simulink library "Lib_CanCommunication"  (R2019b)
settings: Solver=VariableStepAuto  StartTime=0.0  StopTime=10.0  RelTol=1e-3
PostLoadFcn:
  | , if any(exist('dsrtsu_mdlpostloadfcn', 'file') == [2, 3, 6]), try dsrtsu_mdlpostloadfcn('Execute', bdroot); catch fprintf('Error in PostLoadFcn (dsrtsu_mdlpostloadfcn) for model "%s":\n %s\n', bdroot, lasterr); end, end,
undefined symbols (not defined in the file): Counter, CRC, default_customer_can_bus, default_vehicle_state_bus, LateralAcceleration, LongitudinalAcceleration, Motion, Powertrain_1, Steering, steering_angle_range_rad_to_steering_wheel_angle_range_deg_gain, SteeringWheelAngle, SteeringWheelAngleSign, SteeringWheelSpeed, SteeringWheelSpeedSign, SteeringWheelTorque, SteeringWheelTorqueSign, VehicleVelocity, YawRate, YawRateSign
libraries: rtican x8, simulink x6
(part 1 of 3)
settings Model: DSRTSU_INTERNAL_RTI_VER=550  DSRTSU_INTERNAL_RTI_TYPE=rti1401  RTICANMMDATA=struct('GeneralSetupData',struct('modelroot','C:\fav\stack\src\autobox\Simulink\Models','generalsettings',struct('filesettings',struct('destfolder',struct('Name','RTICANMM_FILES','Check',1),'buildfolder',struct('Name','.','Check',1),'AbsDestfolder',struct('Name','C:\fav\stack\src\autobox\Simulink\Models\RTICANMM_FILES'),'AbsBuildfolder',struct('Name','C:\fav\stack\src\autobox\Simulink\Models'))),'options',struct('addpaths',1,'rmpaths',1,'addtrcexclusion',logical(1),'cannavigator',struct('checkmonitoring',0),'show_usrtrc',0,'use_usrtrc',0),'advanced',struct('options',[1 1 1 1 1 1 1 1 1 1 1 1 1 1 1 1 1 1 1 1 1 1 1 1 1 1 1 1 1 1 1 1 1 1 1 1 1 1 1 1 1 1 1 1 1 1 1 1 1 1 1 1 1 1 1 1 1 1 1 1 1 1 1 1 1 1 1 1 1 1 1 1 1 1 1 1 1 1 1 1 1 1 1 1 1 1 1 1 1 1 1 1 1 1 1 1 1 1 1 1]),'MPSetup',{{}},'modelname','Lib_CanCommunication','block','Lib_CanCommunication'))  DSRTSU_INTERNAL_RTIFPGA=150  Creator=bernhard  LastModifiedBy=kessler
settings DataIOCC: ReturnWorkspaceOutputs=off
settings DebuggingCC: ArithmeticOperatorsInVariantConditions=warning
settings SFSimCC: SimUseLocalCustomCode=off  CustomCodeUndefinedFunction=UseInterfaceOnly
settings RTWCC: RTWUseLocalCustomCode=off

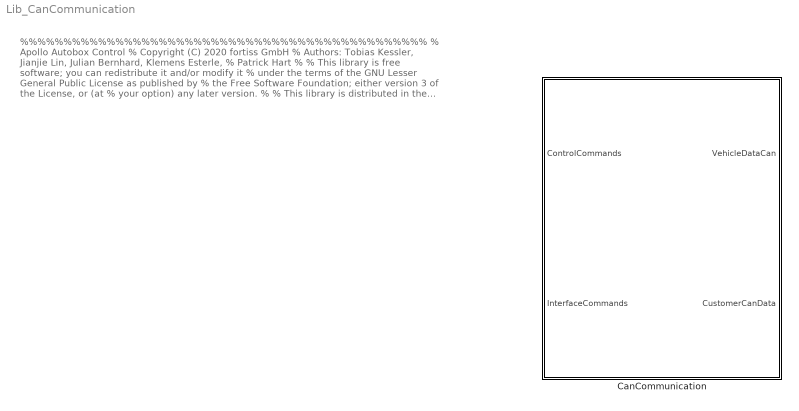
== system Lib_CanCommunication ==
  note: %%%%%%%%%%%%%%%%%%%%%%%%%%%%%%%%%%%%%%%%%%%%%%%
      | % Apollo Autobox Control
      | % Copyright (C) 2020 fortiss GmbH
      | % Authors: Tobias Kessler, Jianjie Lin, Julian Bernhard, Klemens Esterle,
      | % Patrick Hart
      | %
      | % This library is free software; you can redistribute it and/or modify it
      | % under the terms of the GNU Lesser General Public License as published by
      | % the Free Software Foundation; either version 3 of the License, or (at
      | % your option) any later version.
      | %
      | % This library is distributed in the hope that it will be useful, but
      | % WITHOUT ANY WARRANTY; without even the implied warranty of
      | % MERCHANTABILITY or FITNESS FOR A PARTICULAR PURPOSE. See the GNU Lesser
      | % General Public License for more details.
      | %
      | % You should have received a copy of the GNU Lesser General Public License
      | % along with this library; if not, write to the Free Software Foundation,
      | % Inc., 51 Franklin Street, Fifth Floor, Boston, MA 02110-1301, USA.
      | %%%%%%%%%%%%%%%%%%%%%%%%%%%%%%%%%%%%%%%%%%%%%%%
  CanCommunication : Subsystem

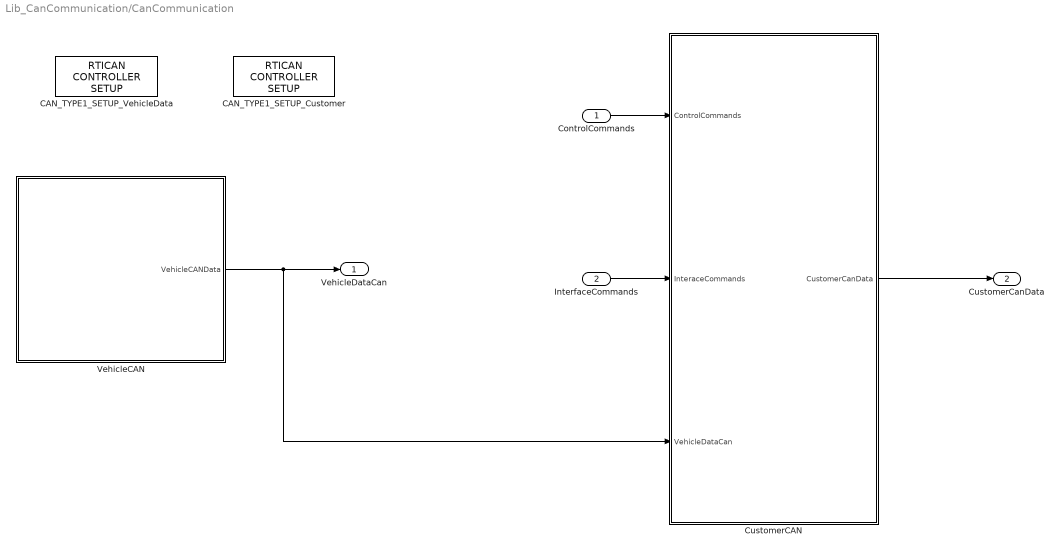
== system Lib_CanCommunication/CanCommunication ==
  ControlCommands : Inport  OutDataTypeStr=Bus: ControlCommands
  InterfaceCommands : Inport  Port=2  OutDataTypeStr=Bus: InterfaceCommands
  CAN_TYPE1_SETUP_Customer : rtican/RTICAN CONTROLLER SETUP   Reserved1=[]  Reserved2=[]  Reserved3=[]  Reserved4=[]  AcceptanceMask=[]  ArbitrationField=[]  Parameters=[]  SFcnRTICANSettings=[]  MS_Struct=[]  BoardTypeNo=[]  BoardNo=[]  ChannelNo=[]  DialogFcn=[]  UnitName=[]  Revision=[]  UnitValues=[]  DSProperties=struct('RTI',struct('Version',uint32(12),'BlockType',struct('isSLSource',uint8(0),'isSLSink',uint8(0),'isHWSource',uint8(0),'isHWSink',uint8(0),'isSetup',uint8(1),'isInline',uint8(1),'isNonInline',uint8(0),'isInterrupt',uint8(0),'isChannelwise',uint8(0)),'IOBoardType','RTICAN','UnitType','NON_MESSAGE','Identifier','MASTER','DialogType','ML','BlockSet','RTICAN','SlaveProcessor','CAN'))  RTIBlockInterface=struct('InputPortsWidth',int32(0),'InputPortsActive',0,'OutputPortsWidth',int32(0),'OutputPortsActive',0,'DialogFcn','rtican_master_setup_gui','BlockDisplay',{{['CAN CONTROLLER\n SETUP'],'center'}},'IconTransparency','on','InitLevel',3,'IWork',{{{'',uint32(2)}}},'BlockName',struct('Token',{{'CAN_TYPE','_SETUP_M','_C'}},'BlockParam',{{'BoardTypeNo','BoardNo','ChannelNo'}}),'ParameterTunableNames',{{}})  RTIBlockParameters="struct('BoardTypeNo',{{1,'OFF',[]}},'BoardNo',{{1,'ON',[1 16]}},'ChannelNo',{{1,'ON',[1 2]}},'AcceptanceMask',{{0,'OFF',[]}},'ArbitrationField',{{0,'OFF',[]}},'Parameters',{{struct('Config',struct('Baudrate',500,'SampleMode',1,'UsedParamSet',1,'validSettings',1,'isBTRvalues',0,'Advanced',struct('Baudrate',{500,500,500},'Frequency',{24000000,36000000,64000000},'Settings',{struct('SMPL',0,'BRP',0,'NBT',24,'TSEG1',15,'TSEG2',6,'SJW',3,'SP',70),struct('SMPL',0,'BRP',1,'NBT',18,'TSEG1',14,'TSEG2',1,'SJW',1,'SP',88),struct('SMPL',0,'BRP',3,'NBT',16,'TSEG1',12,'TSEG2',1,'SJW',1,'SP',87)},'BTR0',{192,65,67},'BTR1',{111,30,28})),'configType',1,'Options',struct('DataFileSelected',1,'DataFileName',{{'..\\dbc\\customer_can_tfd7-17008-03_fortiss_gte.dbc'}},'DataFileDate',{{['02-Aug-2018 13:38:32']}},'InterfaceFcn','rtican_dbc_file_parser','InterfaceFcnFileName','','LabelConfigType','volatile','AcceptanceMaskSelected',0,'MsgDataType','SgnSpecification','NumType','hex','MaskType','STD','AcceptanceMask',0,'ArbitrationField',0,'UseMultipleMessageAccess',1),'RxReceiveStdOptions',struct('RxServiceStdEnabled',0,'RxServiceStdMsgIdent',1000,'RxServiceStdIdentNumType',1,'RxServiceStdIdentMask',0,'RxServiceStdMaskNumType',1,'RxServiceStdQueueSize',64),'RxReceiveXtdOptions',struct('RxServiceXtdEnabled',0,'RxServiceXtdMsgIdent',1001,'RxServiceXtdIdentNumType',1,'RxServiceXtdIdentMask',0,'RxServiceXtdMaskNumType',1,'RxServiceXtdQueueSize',64),'PartialNetworkingOptions',struct('switchedon',0,'format',1,'idmask',['    XXXXX XXXXXXXX XXXXXXXX XXXXXXXX'],'idcode','0','idfilter','0','datamaskused',0,'datalength',1,'datamask','0x0000000000000000','partialnetworkenable',0),'general',struct('Termination_common',2,'Termination_C252',1,'BusConfigurationRegister',0,'Transceiver','ISO11898','isFromLib',0)),'OFF',[]}},'CCPParameters',{{struct('CRO',struct('Format','STD','NumFormat','hex','Id',1639),'DTO',struct('Format','STD','NumFormat','hex','Id',2017),'StationAdr',struct('NumFormat','hex','Value',57),'StationId',struct('Value',['dSPACE CCP Service']),'Enabled',0),'OFF',[]}},'XCPParameters',{{struct('MASTER',struct('Format','STD','NumFormat','hex','Id',256),'SLAVE',struct('Format','STD','NumFormat','hex','Id',510),'Enabled',0,'PIDTransmissionEnabled',0),'OFF',[]}},'GroupId',{{struct('Group',{{'RTICAN'}},'No',2,'Behavior',{{'EVER'}},'BlockType',{{'SOURCE'}},'NameChangeFlag',1),'OFF',[]}},'SFcnRTICANSettings',{{struct('Baudrate',500,'configType',1,'AdvancedConfig',struct('Frequency',{},'BTR0',{},'BTR1',{}),'UsedParamSet',1,'STDMaskSelected','no','XTDMaskSelected','no','BoardType','DS1','BoardNo',1,'ControllerNo',1,'Transceiver','ISO11898','BusConfigRegister',0,'TerminationRes',-1,'UseMultipleMessageAccess','yes','STDRXSrvcUsed','no','STDRXSrvcMsgId',1000,'STDRXSrvcMsgMask',0,'STDRXSrvcQueueSize',64,'XTDRXSrvcUsed','no','XTDRXSrvcMsgId',1001,'XTDRXSrvcQueueSize',64,'XTDRXSrvcMsgMask',0,'PN_IsPNTransciever',0,'PN_IsPNEnabled',0,'PN_MsgFormat',1,'PN_idcode',0,'PN_idmask',2047,'PN_datamaskused',0,'PN_datalength',0,'PN_datamask',['0xFF, 0xFF, 0xFF, 0xFF, 0xFF, 0xFF, 0xFF, 0xFF']),'OFF',[]}},'SFcnRTICCPSettings',{{struct('CRO',struct('Format','STD','NumFormat','hex','Id',1639),'DTO',struct('Format','STD','NumFormat','hex','Id',2017),'StationAdr',struct('NumFormat','hex','Value',57),'StationId',struct('Value',['dSPACE CCP Service']),'Enabled',0),'OFF',[]}},'SFcnRTIXCPSettings',{{struct('MASTER',struct('Format','STD','NumFormat','hex','Id',256),'SLAVE',struct('Format','STD','NumFormat','hex','Id',510),'Enabled',0,'PIDTransmissionEnabled',0),'OFF',[]}},'TLCFileName',{{'rtican_master_setup','OFF',[]}})"  RTISFcnParameters=struct('SFcnRTICANSettings','struct','SFcnRTICCPSettings','struct','SFcnRTIXCPSettings','struct','AcceptanceMask','int32','ArbitrationField','int32','TLCFileName','char')  RTIBlockParaDefault="struct('BoardTypeNo',4302,'BoardNo',1,'ChannelNo',1,'AcceptanceMask',0,'ArbitrationField',0,'Parameters',struct('Config',struct('Baudrate',500,'SampleMode',1,'UsedParamSet',1,'validSettings',1,'isBTRvalues',0,'Advanced',struct('Frequency',16000000,'BTR0',64,'BTR1',28,'Settings',struct('SMPL',0,'BRP',0,'NBT',16,'TSEG1',12,'TSEG2',1,'SJW',1,'SP',87))),'configType',1,'Options',struct('DataFileSelected',0,'DataFileName',{{['<no datafile support>']}},'DataFileDate',{{''}},'InterfaceFcn','rtican_dbc_file_parser','InterfaceFcnFileName','','LabelConfigType','volatile','AcceptanceMaskSelected',0,'MsgDataType','AllwaysDouble','NumType','hex','MaskType','STD','AcceptanceMask',0,'ArbitrationField',0,'UseMultipleMessageAccess',0),'RxReceiveStdOptions',struct('RxServiceStdEnabled',0,'RxServiceStdMsgIdent',1000,'RxServiceStdIdentNumType',1,'RxServiceStdIdentMask',0,'RxServiceStdMaskNumType',1,'RxServiceStdQueueSize',64),'RxReceiveXtdOptions',struct('RxServiceXtdEnabled',0,'RxServiceXtdMsgIdent',1001,'RxServiceXtdIdentNumType',1,'RxServiceXtdIdentMask',0,'RxServiceXtdMaskNumType',1,'RxServiceXtdQueueSize',64),'PartialNetworkingOptions',struct('switchedon',0,'format',1,'idmask',['    XXXXX XXXXXXXX XXXXXXXX XXXXXXXX'],'idcode','0','idfilter','0','datamaskused',0,'datalength',1,'datamask','0x0000000000000000','partialnetworkenable',0),'general',struct('Termination_common',1,'Termination_C252',1,'BusConfigurationRegister',0,'Transceiver','ISO11898','isFromLib',1)),'CCPParameters',struct('CRO',struct('Format','STD','NumFormat','hex','Id',1639),'DTO',struct('Format','STD','NumFormat','hex','Id',2017),'StationAdr',struct('NumFormat','hex','Value',57),'StationId',struct('Value',['dSPACE CCP Service']),'Enabled',0),'XCPParameters',struct('MASTER',struct('Format','STD','NumFormat','hex','Id',256),'SLAVE',struct('Format','STD','NumFormat','hex','Id',510),'Enabled',0,'PIDTransmissionEnabled',0),'GroupId',struct('Group',{{'RTICAN'}},'No',1,'Behavior',{{'EVER'}},'BlockType',{{'SOURCE'}},'NameChangeFlag',1),'SFcnRTICANSettings',struct('Baudrate',500,'configType',1,'AdvandedConfig',struct('Frequency',16000000,'BTR0','0x40','BTR1','0x1C'),'UsedParamSet',1,'STDMaskSelected','no','XTDMaskSelected','no','BoardType','DS4302','BoardNo',1,'ControllerNo',1,'Transceiver','ISO11898','BusConfigRegister',0,'TerminationRes',120,'UseMultipleMessageAccess','no','STDRXSrvcUsed','no','STDRXSrvcMsgId',1000,'STDRXSrvcMsgMask',0,'STDRXSrvcQueueSize',64,'XTDRXSrvcUsed','no','XTDRXSrvcMsgId',1001,'XTDRXSrvcQueueSize',64,'XTDRXSrvcMsgMask',0),'SFcnRTICCPSettings',struct('CRO',struct('Format','STD','NumFormat','hex','Id',1639),'DTO',struct('Format','STD','NumFormat','hex','Id',2017),'StationAdr',struct('NumFormat','hex','Value',57),'StationId',struct('Value',['dSPACE CCP Service']),'Enabled',0),'SFcnRTIXCPSettings',struct('MASTER',struct('Format','STD','NumFormat','hex','Id',256),'SLAVE',struct('Format','STD','NumFormat','hex','Id',510),'Enabled',0,'PIDTransmissionEnabled',0),'TLCFileName','rtican_master_setup')"
      settings: AttributesFormatString=Group Id: RTICAN2\n  SourceProductName=dSPACE RTI CAN Blockset
  CAN_TYPE1_SETUP_VehicleData : rtican/RTICAN CONTROLLER SETUP   Reserved1=[]  Reserved2=[]  Reserved3=[]  Reserved4=[]  AcceptanceMask=[]  ArbitrationField=[]  Parameters=[]  SFcnRTICANSettings=[]  MS_Struct=[]  BoardTypeNo=[]  BoardNo=[]  ChannelNo=[]  DialogFcn=[]  UnitName=[]  Revision=[]  UnitValues=[]  DSProperties=struct('RTI',struct('Version',uint32(12),'BlockType',struct('isSLSource',uint8(0),'isSLSink',uint8(0),'isHWSource',uint8(0),'isHWSink',uint8(0),'isSetup',uint8(1),'isInline',uint8(1),'isNonInline',uint8(0),'isInterrupt',uint8(0),'isChannelwise',uint8(0)),'IOBoardType','RTICAN','UnitType','NON_MESSAGE','Identifier','MASTER','DialogType','ML','BlockSet','RTICAN','SlaveProcessor','CAN'))  RTIBlockInterface=struct('InputPortsWidth',int32(0),'InputPortsActive',0,'OutputPortsWidth',int32(0),'OutputPortsActive',0,'DialogFcn','rtican_master_setup_gui','BlockDisplay',{{['CAN CONTROLLER\n SETUP'],'center'}},'IconTransparency','on','InitLevel',3,'IWork',{{{'',uint32(2)}}},'BlockName',struct('Token',{{'CAN_TYPE','_SETUP_M','_C'}},'BlockParam',{{'BoardTypeNo','BoardNo','ChannelNo'}}),'ParameterTunableNames',{{}})  RTIBlockParameters="struct('BoardTypeNo',{{1,'OFF',[]}},'BoardNo',{{1,'ON',[1 16]}},'ChannelNo',{{2,'ON',[1 2]}},'AcceptanceMask',{{0,'OFF',[]}},'ArbitrationField',{{0,'OFF',[]}},'Parameters',{{struct('Config',struct('Baudrate',500,'SampleMode',1,'UsedParamSet',1,'validSettings',1,'isBTRvalues',0,'Advanced',struct('Baudrate',{500,500,500},'Frequency',{24000000,36000000,64000000},'Settings',{struct('SMPL',0,'BRP',0,'NBT',24,'TSEG1',15,'TSEG2',6,'SJW',3,'SP',70),struct('SMPL',0,'BRP',1,'NBT',18,'TSEG1',14,'TSEG2',1,'SJW',1,'SP',88),struct('SMPL',0,'BRP',3,'NBT',16,'TSEG1',12,'TSEG2',1,'SJW',1,'SP',87)},'BTR0',{192,65,67},'BTR1',{111,30,28})),'configType',1,'Options',struct('DataFileSelected',1,'DataFileName',{{'..\\dbc\\vehicledata_can_tfd7-17008-03_fortiss_gte.dbc'}},'DataFileDate',{{['02-Aug-2018 13:38:32']}},'InterfaceFcn','rtican_dbc_file_parser','InterfaceFcnFileName','','LabelConfigType','volatile','AcceptanceMaskSelected',0,'MsgDataType','SgnSpecification','NumType','hex','MaskType','STD','AcceptanceMask',0,'ArbitrationField',0,'UseMultipleMessageAccess',1),'RxReceiveStdOptions',struct('RxServiceStdEnabled',0,'RxServiceStdMsgIdent',1000,'RxServiceStdIdentNumType',1,'RxServiceStdIdentMask',0,'RxServiceStdMaskNumType',1,'RxServiceStdQueueSize',64),'RxReceiveXtdOptions',struct('RxServiceXtdEnabled',0,'RxServiceXtdMsgIdent',1001,'RxServiceXtdIdentNumType',1,'RxServiceXtdIdentMask',0,'RxServiceXtdMaskNumType',1,'RxServiceXtdQueueSize',64),'PartialNetworkingOptions',struct('switchedon',0,'format',1,'idmask',['    XXXXX XXXXXXXX XXXXXXXX XXXXXXXX'],'idcode','0','idfilter','0','datamaskused',0,'datalength',1,'datamask','0x0000000000000000','partialnetworkenable',0),'general',struct('Termination_common',2,'Termination_C252',1,'BusConfigurationRegister',0,'Transceiver','ISO11898','isFromLib',0)),'OFF',[]}},'CCPParameters',{{struct('CRO',struct('Format','STD','NumFormat','hex','Id',1639),'DTO',struct('Format','STD','NumFormat','hex','Id',2017),'StationAdr',struct('NumFormat','hex','Value',57),'StationId',struct('Value',['dSPACE CCP Service']),'Enabled',0),'OFF',[]}},'XCPParameters',{{struct('MASTER',struct('Format','STD','NumFormat','hex','Id',256),'SLAVE',struct('Format','STD','NumFormat','hex','Id',510),'Enabled',0,'PIDTransmissionEnabled',0),'OFF',[]}},'GroupId',{{struct('Group',{{'RTICAN'}},'No',1,'Behavior',{{'EVER'}},'BlockType',{{'SOURCE'}},'NameChangeFlag',1),'OFF',[]}},'SFcnRTICANSettings',{{struct('Baudrate',500,'configType',1,'AdvancedConfig',struct('Frequency',{},'BTR0',{},'BTR1',{}),'UsedParamSet',1,'STDMaskSelected','no','XTDMaskSelected','no','BoardType','DS1','BoardNo',1,'ControllerNo',2,'Transceiver','ISO11898','BusConfigRegister',0,'TerminationRes',-1,'UseMultipleMessageAccess','yes','STDRXSrvcUsed','no','STDRXSrvcMsgId',1000,'STDRXSrvcMsgMask',0,'STDRXSrvcQueueSize',64,'XTDRXSrvcUsed','no','XTDRXSrvcMsgId',1001,'XTDRXSrvcQueueSize',64,'XTDRXSrvcMsgMask',0,'PN_IsPNTransciever',0,'PN_IsPNEnabled',0,'PN_MsgFormat',1,'PN_idcode',0,'PN_idmask',2047,'PN_datamaskused',0,'PN_datalength',0,'PN_datamask',['0xFF, 0xFF, 0xFF, 0xFF, 0xFF, 0xFF, 0xFF, 0xFF']),'OFF',[]}},'SFcnRTICCPSettings',{{struct('CRO',struct('Format','STD','NumFormat','hex','Id',1639),'DTO',struct('Format','STD','NumFormat','hex','Id',2017),'StationAdr',struct('NumFormat','hex','Value',57),'StationId',struct('Value',['dSPACE CCP Service']),'Enabled',0),'OFF',[]}},'SFcnRTIXCPSettings',{{struct('MASTER',struct('Format','STD','NumFormat','hex','Id',256),'SLAVE',struct('Format','STD','NumFormat','hex','Id',510),'Enabled',0,'PIDTransmissionEnabled',0),'OFF',[]}},'TLCFileName',{{'rtican_master_setup','OFF',[]}})"  RTISFcnParameters=struct('SFcnRTICANSettings','struct','SFcnRTICCPSettings','struct','SFcnRTIXCPSettings','struct','AcceptanceMask','int32','ArbitrationField','int32','TLCFileName','char')  RTIBlockParaDefault="struct('BoardTypeNo',4302,'BoardNo',1,'ChannelNo',1,'AcceptanceMask',0,'ArbitrationField',0,'Parameters',struct('Config',struct('Baudrate',500,'SampleMode',1,'UsedParamSet',1,'validSettings',1,'isBTRvalues',0,'Advanced',struct('Frequency',16000000,'BTR0',64,'BTR1',28,'Settings',struct('SMPL',0,'BRP',0,'NBT',16,'TSEG1',12,'TSEG2',1,'SJW',1,'SP',87))),'configType',1,'Options',struct('DataFileSelected',0,'DataFileName',{{['<no datafile support>']}},'DataFileDate',{{''}},'InterfaceFcn','rtican_dbc_file_parser','InterfaceFcnFileName','','LabelConfigType','volatile','AcceptanceMaskSelected',0,'MsgDataType','AllwaysDouble','NumType','hex','MaskType','STD','AcceptanceMask',0,'ArbitrationField',0,'UseMultipleMessageAccess',0),'RxReceiveStdOptions',struct('RxServiceStdEnabled',0,'RxServiceStdMsgIdent',1000,'RxServiceStdIdentNumType',1,'RxServiceStdIdentMask',0,'RxServiceStdMaskNumType',1,'RxServiceStdQueueSize',64),'RxReceiveXtdOptions',struct('RxServiceXtdEnabled',0,'RxServiceXtdMsgIdent',1001,'RxServiceXtdIdentNumType',1,'RxServiceXtdIdentMask',0,'RxServiceXtdMaskNumType',1,'RxServiceXtdQueueSize',64),'PartialNetworkingOptions',struct('switchedon',0,'format',1,'idmask',['    XXXXX XXXXXXXX XXXXXXXX XXXXXXXX'],'idcode','0','idfilter','0','datamaskused',0,'datalength',1,'datamask','0x0000000000000000','partialnetworkenable',0),'general',struct('Termination_common',1,'Termination_C252',1,'BusConfigurationRegister',0,'Transceiver','ISO11898','isFromLib',1)),'CCPParameters',struct('CRO',struct('Format','STD','NumFormat','hex','Id',1639),'DTO',struct('Format','STD','NumFormat','hex','Id',2017),'StationAdr',struct('NumFormat','hex','Value',57),'StationId',struct('Value',['dSPACE CCP Service']),'Enabled',0),'XCPParameters',struct('MASTER',struct('Format','STD','NumFormat','hex','Id',256),'SLAVE',struct('Format','STD','NumFormat','hex','Id',510),'Enabled',0,'PIDTransmissionEnabled',0),'GroupId',struct('Group',{{'RTICAN'}},'No',1,'Behavior',{{'EVER'}},'BlockType',{{'SOURCE'}},'NameChangeFlag',1),'SFcnRTICANSettings',struct('Baudrate',500,'configType',1,'AdvandedConfig',struct('Frequency',16000000,'BTR0','0x40','BTR1','0x1C'),'UsedParamSet',1,'STDMaskSelected','no','XTDMaskSelected','no','BoardType','DS4302','BoardNo',1,'ControllerNo',1,'Transceiver','ISO11898','BusConfigRegister',0,'TerminationRes',120,'UseMultipleMessageAccess','no','STDRXSrvcUsed','no','STDRXSrvcMsgId',1000,'STDRXSrvcMsgMask',0,'STDRXSrvcQueueSize',64,'XTDRXSrvcUsed','no','XTDRXSrvcMsgId',1001,'XTDRXSrvcQueueSize',64,'XTDRXSrvcMsgMask',0),'SFcnRTICCPSettings',struct('CRO',struct('Format','STD','NumFormat','hex','Id',1639),'DTO',struct('Format','STD','NumFormat','hex','Id',2017),'StationAdr',struct('NumFormat','hex','Value',57),'StationId',struct('Value',['dSPACE CCP Service']),'Enabled',0),'SFcnRTIXCPSettings',struct('MASTER',struct('Format','STD','NumFormat','hex','Id',256),'SLAVE',struct('Format','STD','NumFormat','hex','Id',510),'Enabled',0,'PIDTransmissionEnabled',0),'TLCFileName','rtican_master_setup')"
      settings: AttributesFormatString=Group Id: RTICAN1\n  SourceProductName=dSPACE RTI CAN Blockset
  CustomerCAN : Subsystem
  VehicleCAN : Subsystem
  VehicleDataCan : Outport  OutDataTypeStr=Bus: vehicle_data_can_bus  VectorParamsAs1DForOutWhenUnconnected=off
  CustomerCanData : Outport  Port=2  OutDataTypeStr=Bus: customer_can_bus  VectorParamsAs1DForOutWhenUnconnected=off
  wires:
  VehicleCAN/1(VehicleCANData) -> VehicleDataCan/1, CustomerCAN/3(VehicleDataCan)
  CustomerCAN/1(CustomerCanData) -> CustomerCanData/1
  ControlCommands/1 -> CustomerCAN/1(ControlCommands)
  InterfaceCommands/1 -> CustomerCAN/2(InteraceCommands)

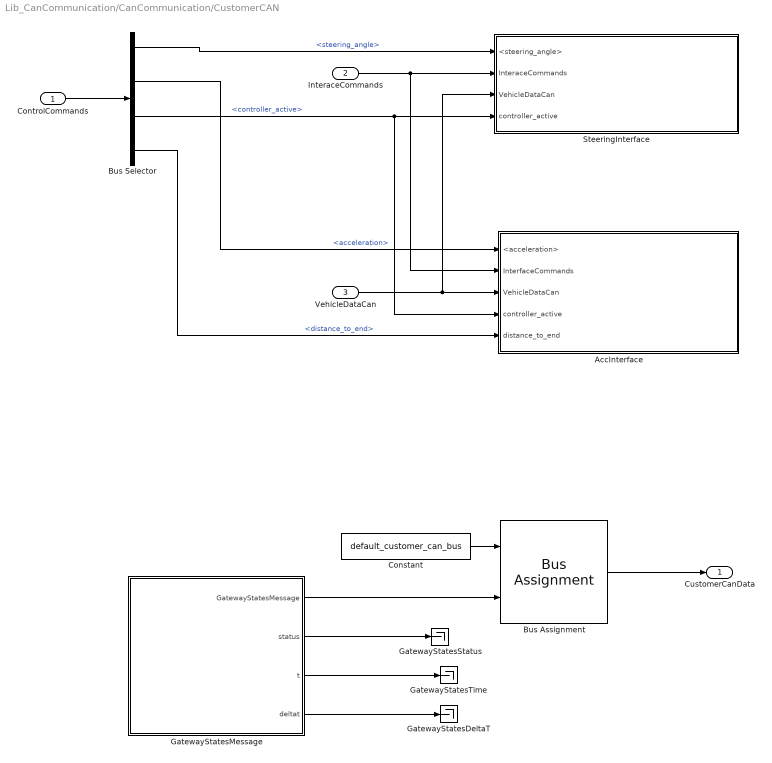
== system Lib_CanCommunication/CanCommunication/CustomerCAN ==
  ControlCommands : Inport  OutDataTypeStr=Bus: ControlCommands
  InteraceCommands : Inport  Port=2  OutDataTypeStr=Bus: InterfaceCommands
  VehicleDataCan : Inport  Port=3
  AccInterface : Subsystem
  Bus Assignment : BusAssignment  AssignedSignals=Gateway_States
  Bus Selector : BusSelector  OutputSignals=steering_angle,acceleration,controller_active,distance_to_end
  Constant : Constant  Value=default_customer_can_bus  OutDataTypeStr=Bus: customer_can_bus
  GatewayStatesDeltaT : Terminator
  GatewayStatesMessage : Subsystem
  GatewayStatesStatus : Terminator
  GatewayStatesTime : Terminator
  SteeringInterface : Subsystem
  CustomerCanData : Outport  VectorParamsAs1DForOutWhenUnconnected=off
  wires:
  Bus Selector/4 -> AccInterface/5(distance_to_end)  "<distance_to_end>"
  Bus Selector/1 -> SteeringInterface/1(<steering_angle>)  "<steering_angle>"
  Bus Selector/2 -> AccInterface/1(<acceleration>)  "<acceleration>"
  Bus Selector/3 -> SteeringInterface/4(controller_active), AccInterface/4(controller_active)  "<controller_active>"
  VehicleDataCan/1 -> AccInterface/3(VehicleDataCan), SteeringInterface/3(VehicleDataCan)
  Constant/1 -> Bus Assignment/1
  Bus Assignment/1 -> CustomerCanData/1
  ControlCommands/1 -> Bus Selector/1
  InteraceCommands/1 -> SteeringInterface/2(InteraceCommands), AccInterface/2(InterfaceCommands)
  GatewayStatesMessage/2(status) -> GatewayStatesStatus/1
  GatewayStatesMessage/3(t) -> GatewayStatesTime/1
  GatewayStatesMessage/4(deltat) -> GatewayStatesDeltaT/1
  GatewayStatesMessage/1(GatewayStatesMessage) -> Bus Assignment/2

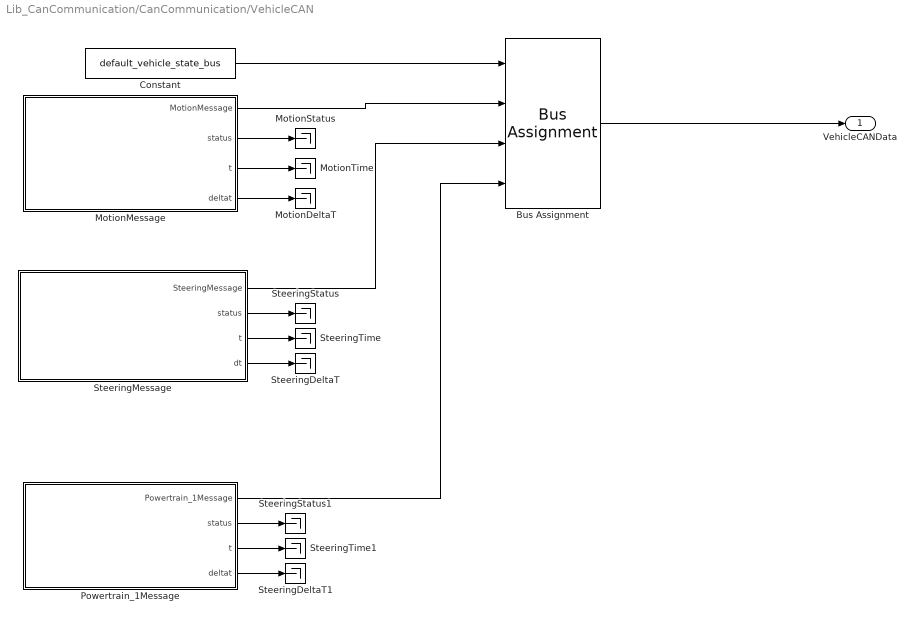
== system Lib_CanCommunication/CanCommunication/VehicleCAN ==
  Bus Assignment : BusAssignment  AssignedSignals=Motion,Steering,Powertrain_1
  Constant : Constant  Value=default_vehicle_state_bus  OutDataTypeStr=Bus: vehicle_data_can_bus
  MotionDeltaT : Terminator
  MotionMessage : Subsystem
  MotionStatus : Terminator
  MotionTime : Terminator
  Powertrain_1Message : Subsystem
  SteeringDeltaT : Terminator
  SteeringDeltaT1 : Terminator
  SteeringMessage : Subsystem
  SteeringStatus : Terminator
  SteeringStatus1 : Terminator
  SteeringTime : Terminator
  SteeringTime1 : Terminator
  VehicleCANData : Outport  VectorParamsAs1DForOutWhenUnconnected=off
  wires:
  Powertrain_1Message/1(Powertrain_1Message) -> Bus Assignment/4
  Powertrain_1Message/4(deltat) -> SteeringDeltaT1/1
  Powertrain_1Message/2(status) -> SteeringStatus1/1
  Powertrain_1Message/3(t) -> SteeringTime1/1
  SteeringMessage/3(t) -> SteeringTime/1
  MotionMessage/2(status) -> MotionStatus/1
  MotionMessage/4(deltat) -> MotionDeltaT/1
  SteeringMessage/2(status) -> SteeringStatus/1
  SteeringMessage/4(dt) -> SteeringDeltaT/1
  MotionMessage/3(t) -> MotionTime/1
  Bus Assignment/1 -> VehicleCANData/1
  MotionMessage/1(MotionMessage) -> Bus Assignment/2
  Constant/1 -> Bus Assignment/1
  SteeringMessage/1(SteeringMessage) -> Bus Assignment/3

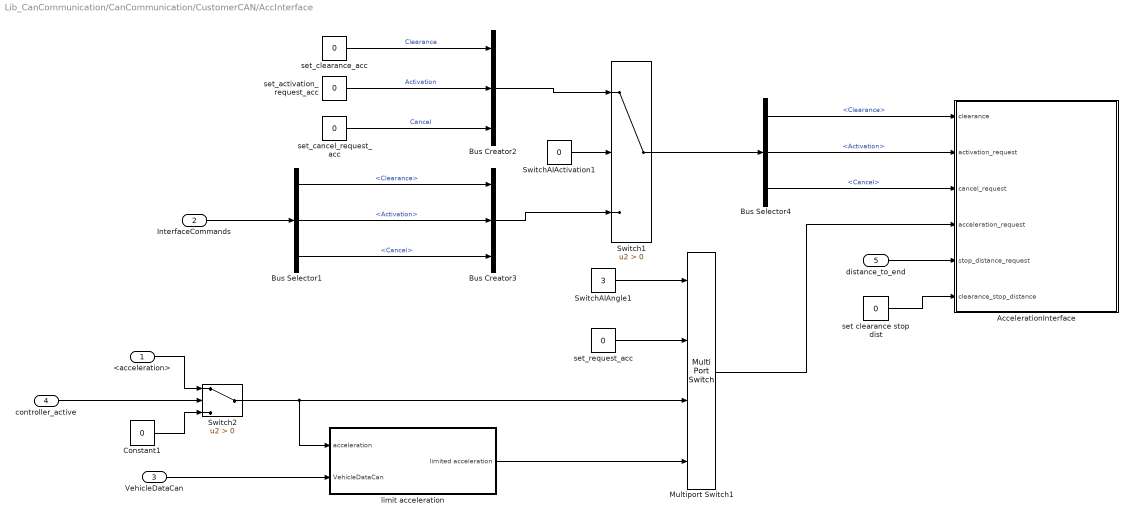
== system Lib_CanCommunication/CanCommunication/CustomerCAN/AccInterface ==
  <acceleration> : Inport
  InterfaceCommands : Inport  Port=2
  VehicleDataCan : Inport  Port=3
  controller_active : Inport  Port=4
  distance_to_end : Inport  Port=5
  AccelerationInterface : Subsystem
  Bus Creator2 : BusCreator  Inputs=3
  Bus Creator3 : BusCreator  Inputs=3
  Bus Selector1 : BusSelector  OutputSignals=AccelerationInterfaceCommands.Clearance,AccelerationInterfaceCommands.Activation,AccelerationInterfaceCommands.Cancel
  Bus Selector4 : BusSelector  OutputSignals=Clearance,Activation,Cancel
  Constant1 : Constant  Value=0
  Multiport Switch1 : MultiPortSwitch
  Switch1 : Switch  Criteria=u2 > Threshold
  Switch2 : Switch  Criteria=u2 > Threshold
  SwitchAIActivation1 : Constant  Value=0
  SwitchAIAngle1 : Constant  Value=3
  limit acceleration : Subsystem
  set clearance stop dist : Constant  Value=0  OutDataTypeStr=boolean
  set_activation_request_acc : Constant  Value=0  OutDataTypeStr=boolean
  set_cancel_request_acc : Constant  Value=0  OutDataTypeStr=boolean
  set_clearance_acc : Constant  Value=0  OutDataTypeStr=boolean
  set_request_acc : Constant  Value=0
  wires:
  set clearance stop dist/1 -> AccelerationInterface/6(clearance_stop_distance)
  distance_to_end/1 -> AccelerationInterface/5(stop_distance_request)
  controller_active/1 -> Switch2/2
  <acceleration>/1 -> Switch2/1
  Constant1/1 -> Switch2/3
  set_request_acc/1 -> Multiport Switch1/2
  Bus Selector1/2 -> Bus Creator3/2  "<Activation>"
  Bus Creator3/1 -> Switch1/3
  set_clearance_acc/1 -> Bus Creator2/1  "Clearance"
  Bus Selector4/3 -> AccelerationInterface/3(cancel_request)  "<Cancel>"
  Bus Selector1/1 -> Bus Creator3/1  "<Clearance>"
  Bus Selector4/1 -> AccelerationInterface/1(clearance)  "<Clearance>"
  Multiport Switch1/1 -> AccelerationInterface/4(acceleration_request)
  SwitchAIActivation1/1 -> Switch1/2
  set_activation_request_acc/1 -> Bus Creator2/2  "Activation"
  Bus Creator2/1 -> Switch1/1
  Bus Selector4/2 -> AccelerationInterface/2(activation_request)  "<Activation>"
  Switch1/1 -> Bus Selector4/1
  Bus Selector1/3 -> Bus Creator3/3  "<Cancel>"
  set_cancel_request_acc/1 -> Bus Creator2/3  "Cancel"
  SwitchAIAngle1/1 -> Multiport Switch1/1
  limit acceleration/1(limited acceleration) -> Multiport Switch1/4
  InterfaceCommands/1 -> Bus Selector1/1
  VehicleDataCan/1 -> limit acceleration/2(VehicleDataCan)
  Switch2/1 -> limit acceleration/1(acceleration), Multiport Switch1/3

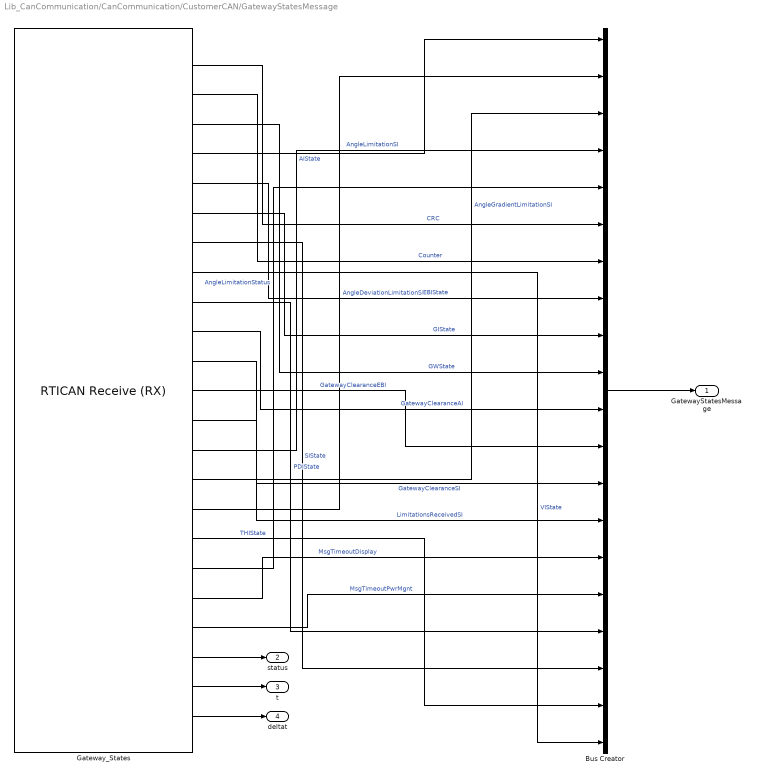
== system Lib_CanCommunication/CanCommunication/CustomerCAN/GatewayStatesMessage ==
  Bus Creator : BusCreator  Inputs=20  OutDataTypeStr=Bus: Gateway_States  NonVirtualBus=on
  Gateway_States : rtican/RTICAN Receive (RX)   Reserved1=[]  Reserved2=[]  Reserved3=[]  Reserved4=[]  SfcnMessage=[]  Msg_Struct=[]  BoardTypeNo=[]  BoardNo=[]  ChannelNo=[]  Parameters=[]  DialogFcn=[]  UnitName=[]  Revision=[]  UnitValues=[]  DSProperties=struct('RTI',struct('Version',uint32(5),'BlockType',struct('isSLSource',uint8(1),'isSLSink',uint8(1),'isHWSource',uint8(0),'isHWSink',uint8(0),'isSetup',uint8(0),'isInline',uint8(1),'isNonInline',uint8(0),'isInterrupt',uint8(0),'isChannelwise',uint8(0)),'IOBoardType','RTICAN','UnitType','MESSAGE','Identifier','RX','DialogType','MSVC','BlockSet','RTICAN','SlaveProcessor','CAN'))  RTIBlockInterface=struct('OutputPortsWidth',int32([1 1 1 1 1 1 1 1 1 1 1 1 1 1 1 1 1 1 1 1 1 1 1]),'OutputPortsActive',ones(1,23),'OutputPortsName',{{'CRC','Counter','GWState','AIState','EBIState','GIState','SIState','VIState','PDIState','GatewayClearanceAI','GatewayClearanceSI','GatewayClearanceEBI','LimitationsReceivedSI','AngleLimitationSI','AngleGradientLimitationSI','AngleDeviationLimitationSI','THIState','AngleLimitationStatus','MsgTimeoutDisplay','MsgTimeoutPwrMgnt',['RX status'],['RX time'],['RX delta time']}},'OutputPortsDataType',{{'SS_UINT8','SS_UINT8','SS_UINT8','SS_UINT8','SS_UINT8','SS_UINT8','SS_UINT8','SS_UINT8','SS_UINT8','SS_BOOLEAN','SS_BOOLEAN','SS_BOOLEAN','SS_UINT8','SS_BOOLEAN','SS_BOOLEAN','SS_BOOLEAN','SS_UINT8','SS_BOOLEAN','SS_BOOLEAN','SS_BOOLEAN','SS_DOUBLE','SS_DOUBLE','SS_DOUBLE'}},'OutputPortsLabel',{{'CRC','Counter','GWState','AIState','EBIState','GIState','SIState','VIState','PDIState','GatewayClearanceAI','GatewayClearanceSI','GatewayClearanceEBI','LimitationsReceivedSI','AngleLimitationSI','AngleGradientLimitationSI','AngleDeviationLimitationSI','THIState','AngleLimitationStatus','MsgTimeoutDisplay','MsgTimeoutPwrMgnt','','',''}},'OutputPortsLabelMode','ON','InputPortsWidth',int32(0),'InputPortsActive',0,'DialogFcn','rtican_message_interface_gui','BlockDisplay',{{'','center'}},'IconTransparency','on','ParameterTunableNames',{{}},'InitLevel',3,'BlockName',struct('Token',{{'Gateway_States'}}),'SampleTime',{{-1}},'TriggerPort',{{'none'}},'EnablePort',{{'none'}})  RTIBlockParameters=struct('BoardTypeNo',{{1,'OFF',[]}},'BoardNo',{{1,'ON',[1 16]}},'ChannelNo',{{1,'ON',[1 2]}},'Parameters',{{struct('DataFileSupport',struct('DataFileSelectedMaster',1,'DataFileSelectedLocal',1,'DataFileName','c:\users\esterle\documents\repositories\stack\src\autobox\simulink\dbc\customer_can_tfd7-17008-03_fortiss_gte.dbc|','DataFileDate',{{{['11-Jul-2018 11:13:29']},{['11-Jul-2018 11:13:29']}}},'SelectedFile','..\dbc\customer_can_tfd7-17008-03_fortiss_gte.dbc'),'Options',struct('StatusSelected',1,'TimeSelected',1,'DeltaTimeSelected',1,'BytePortSelected',0,'MessageLengthSelected',0,'TriggerPort',struct('Selected',0,'TriggerType',0),'UserCoding',struct('Selected',0,'InterfaceFile','UserDecodingFile','FcnName','UserDecodeFcn','InportSelected',0,'InportWidth',1,'OutportSelected',0,'OutportWidth',1),'EnablePortSelected',0,'SignalOnPortnameSelected',1,'UseRXService',0),'Message',struct('MsgOnBlocknameSelected',1,'MsgName','Gateway_States','MsgIdFormat',0,'MsgId',336,'MsgLength',8,'NumSignals',20,'SampleTime',-1,'Signal',struct('SgnName',{'CRC','Counter','GWState','AIState','EBIState','GIState','SIState','VIState','PDIState','GatewayClearanceAI','GatewayClearanceSI','GatewayClearanceEBI','LimitationsReceivedSI','AngleLimitationSI','AngleGradientLimitationSI','AngleDeviationLimitationSI','THIState','AngleLimitationStatus','MsgTimeoutDisplay','MsgTimeoutPwrMgnt'},'SgnStartBit',{0,8,12,16,20,24,28,32,36,40,41,42,43,45,46,47,48,60,61,62},'SgnLength',{8,4,4,4,4,4,4,4,4,1,1,1,2,1,1,1,4,1,1,1},'SgnType',{0,0,0,0,0,0,0,0,0,0,0,0,0,0,0,0,0,0,0,0},'ModeValue',{-1,-1,-1,-1,-1,-1,-1,-1,-1,-1,-1,-1,-1,-1,-1,-1,-1,-1,-1,-1},'DataType',{0,0,0,0,0,0,0,0,0,0,0,0,0,0,0,0,0,0,0,0},'ByteLayout',{0,0,0,0,0,0,0,0,0,0,0,0,0,0,0,0,0,0,0,0},'Factor',{1,1,1,1,1,1,1,1,1,1,1,1,1,1,1,1,1,1,1,1},'Offset',{0,0,0,0,0,0,0,0,0,0,0,0,0,0,0,0,0,0,0,0},'SgnComment',{{['Checksum for GW States message CRC = Byte1 XOR Byte2 XOR Byte3 XOR Byte4 XOR Byte5 XOR Byte6 XOR Byte7.']},{['Counter for GW States message, incremented with every transmittal and periodically running from 0 to 15.']},{['General state of gateway.']},{['State of the Acceleration Interface. ']},{['State of the Emergency Brake Interface.']},{['State of the Gear Shift Interface.']},{['State of the Steering Interface.']},{['State of the Vehicle Interface.']},{['State of the Park Deceleration Interface.']},{['Internal clearance signal of the Acceleration Interface (key switch & interface clearance).']},{['Internal clearance signal of the Steering Interface (key switch & interface clearance).']},{['Internal clearance signal of the Emergency Brake Interface (key switch & interface clearance).']},{['Steering wheel angle limitations have been received correctly. ']},{['Steering wheel angle is limited. ']},{['Steering wheel angle gradient is limited. ']},{['Steering wheel angle deviation is limited. ']},{['State of the Throttle Interface.']},{['Status of steering wheel angle limitation characteristic (for future use).']},{['Indicates timeout of display status message.']},{['Indicates timeout of power management status message.']}},'SgnUnit',{'-','-','-','-','-','-','-','-','-','-','-','-','-','-','-','-','-','-','-','-'},'Min',{0,0,0,0,0,0,0,0,0,0,0,0,0,0,0,0,0,0,0,0},'Max',{255,15,15,15,15,15,15,15,15,1,1,1,3,1,1,1,15,1,1,1},'SLDataType',{'SS_UINT8','SS_UINT8','SS_UINT8','SS_UINT8','SS_UINT8','SS_UINT8','SS_UINT8','SS_UINT8','SS_UINT8','SS_BOOLEAN','SS_BOOLEAN','SS_BOOLEAN','SS_UINT8','SS_BOOLEAN','SS_BOOLEAN','SS_BOOLEAN','SS_UINT8','SS_BOOLEAN','SS_BOOLEAN','SS_BOOLEAN'}),'MsgIdNumFormat',0,'MsgComment',{{['Information about the Gateway states. ']}}),'Version',1.2,'general',struct('isFromLib',0)),'OFF',[]}},'GroupId',{{struct('Group',{{'RTICAN'}},'No',2,'Behavior',{{'NAMECHANGE'}},'BlockType',{{'SINK'}},'NameChangeFlag',0),'OFF',[]}},'SFcnRTICANMessage',{{struct('MsgType','RX','SFcnPortType','Scalar','MsgName','Gateway_States','MsgIdFormat','STD','MsgId',336,'MsgLength',8,'NumSignals',20,'SampleTime',-1,'Signal',struct('SgnName',{'CRC','Counter','GWState','AIState','EBIState','GIState','SIState','VIState','PDIState','GatewayClearanceAI','GatewayClearanceSI','GatewayClearanceEBI','LimitationsReceivedSI','AngleLimitationSI','AngleGradientLimitationSI','AngleDeviationLimitationSI','THIState','AngleLimitationStatus','MsgTimeoutDisplay','MsgTimeoutPwrMgnt'},'SgnStartBit',{0,8,12,16,20,24,28,32,36,40,41,42,43,45,46,47,48,60,61,62},'SgnLength',{8,4,4,4,4,4,4,4,4,1,1,1,2,1,1,1,4,1,1,1},'SgnType',{'standard','standard','standard','standard','standard','standard','standard','standard','standard','standard','standard','standard','standard','standard','standard','standard','standard','standard','standard','standard'},'ModeValue',{-1,-1,-1,-1,-1,-1,-1,-1,-1,-1,-1,-1,-1,-1,-1,-1,-1,-1,-1,-1},'DataType',{['unsigned int'],['unsigned int'],['unsigned int'],['unsigned int'],['unsigned int'],['unsigned int'],['unsigned int'],['unsigned int'],['unsigned int'],['unsigned int'],['unsigned int'],['unsigned int'],['unsigned int'],['unsigned int'],['unsigned int'],['unsigned int'],['unsigned int'],['unsigned int'],['unsigned int'],['unsigned int']},'ByteLayout',{['little endian'],['little endian'],['little endian'],['little endian'],['little endian'],['little endian'],['little endian'],['little endian'],['little endian'],['little endian'],['little endian'],['little endian'],['little endian'],['little endian'],['little endian'],['little endian'],['little endian'],['little endian'],['little endian'],['little endian']},'Factor',{1,1,1,1,1,1,1,1,1,1,1,1,1,1,1,1,1,1,1,1},'Offset',{0,0,0,0,0,0,0,0,0,0,0,0,0,0,0,0,0,0,0,0},'SLDataType',{'SS_UINT8','SS_UINT8','SS_UINT8','SS_UINT8','SS_UINT8','SS_UINT8','SS_UINT8','SS_UINT8','SS_UINT8','SS_BOOLEAN','SS_BOOLEAN','SS_BOOLEAN','SS_UINT8','SS_BOOLEAN','SS_BOOLEAN','SS_BOOLEAN','SS_UINT8','SS_BOOLEAN','SS_BOOLEAN','SS_BOOLEAN'}),'StatusSelected','yes','TimeSelected','yes','DeltaTimeSelected','yes','BytePortSelected','no','MessageLengthSelected','no','TriggerPort',struct('Selected','no','TriggerType',0),'UserCoding',struct('Selected','no','InterfaceFile','UserDecodingFile','FcnName','UserDecodeFcn','InportSelected','no','InportWidth',1,'OutportSelected','no','OutportWidth',1),'EnablePortSelected','no','UseRXService','no','BoardType','DS1','BoardNo',1,'ControllerNo',1),'OFF',[]}},'TLCFileName',{{'rtican_rx_message','OFF',[]}})  RTISFcnParameters=struct('SFcnRTICANMessage','struct','TLCFileName','char')  RTIBlockParaDefault=struct('BoardTypeNo',4302,'BoardNo',1,'ChannelNo',1,'Parameters',struct('DataFileSupport',struct('DataFileSelectedMaster',0,'DataFileSelectedLocal',0,'DataFileName','','DataFileDate','','SelectedFile',['<no file selected>']),'Options',struct('StatusSelected',1,'TimeSelected',1,'DeltaTimeSelected',1,'BytePortSelected',0,'MessageLengthSelected',0,'TriggerPort',struct('Selected',0,'TriggerType','rising'),'UserCoding',struct('Selected',0,'InterfaceFile','UserDecodingFile','FcnName','UserDecodeFcn','InportSelected',0,'InportWidth',1,'OutportSelected',0,'OutportWidth',1),'EnablePortSelected',0,'SignalOnPortnameSelected',1,'UseRXService',0),'Message',struct('MsgOnBlocknameSelected',0,'MsgName',['RX Message'],'MsgIdFormat',0,'MsgId',100,'MsgLength',8,'NumSignals',1,'SampleTime',-1,'Signal',struct('SgnName',['RX signal'],'SgnStartBit',0,'SgnLength',8,'SgnType',0,'ModeValue',-1,'DataType',0,'SLDataType','SS_DOUBLE','ByteLayout',0,'Factor',1,'Offset',0,'Min',0,'Max',255,'SgnComment',{{}},'SgnUnit',''),'MsgIdNumFormat',0,'MsgComment',{{''}}),'Version',1.2,'general',struct('isFromLib',1)),'GroupId',struct('Group',{{'RTICAN'}},'No',1,'Behavior',{{'NAMECHANGE'}},'BlockType',{{'SINK'}},'NameChangeFlag',0),'SFcnRTICANMessage',struct('MsgType','RX','MsgName',['RX Message'],'MsgIdFormat','STD','MsgId',100,'MsgLength',8,'NumSignals',1,'SampleTime',-1,'Signal',struct('SgnName',['RX signal'],'SgnStartBit',0,'SgnLength',8,'SgnType','standard','ModeValue',-1,'DataType',['unsigned int'],'ByteLayout',['little endian'],'SLDataType','SS_DOUBLE','Factor',1,'Offset',0),'StatusSelected','yes','TimeSelected','yes','DeltaTimeSelected','yes','BytePortSelected','no','MessageLengthSelected','no','EnablePortSelected','no','UserCoding',struct('Selected','no','InterfaceFile','UserDecodingFile','FcnName','UserDecodeFcn','InportSelected','no','InportWidth',1,'OutportSelected','no','OutportWidth',1),'TriggerPort',struct('Selected','no','TriggerType','rising'),'UseRXService','no','BoardType','DS4302','BoardNo',1,'ControllerNo',1,'SFcnPortType','Scalar'),'TLCFileName','rtican_rx_message')
      settings: AttributesFormatString=Group Id: RTICAN2\n  SourceProductName=dSPACE RTI CAN Blockset
  GatewayStatesMessage : Outport  VectorParamsAs1DForOutWhenUnconnected=off
  status : Outport  Port=2  VectorParamsAs1DForOutWhenUnconnected=off
  t : Outport  Port=3  VectorParamsAs1DForOutWhenUnconnected=off
  deltat : Outport  Port=4  VectorParamsAs1DForOutWhenUnconnected=off
  wires:
  Gateway_States/22 -> t/1
  Bus Creator/1 -> GatewayStatesMessage/1
  Gateway_States/21 -> status/1
  Gateway_States/23 -> deltat/1
  Gateway_States/4 -> Bus Creator/1  "AIState"
  Gateway_States/20 -> Bus Creator/16  "MsgTimeoutPwrMgnt"
  Gateway_States/3 -> Bus Creator/10  "GWState"
  Gateway_States/14 -> Bus Creator/4  "AngleLimitationSI"
  Gateway_States/16 -> Bus Creator/2  "AngleDeviationLimitationSI"
  Gateway_States/18 -> Bus Creator/5  "AngleLimitationStatus"
  Gateway_States/2 -> Bus Creator/7  "Counter"
  Gateway_States/6 -> Bus Creator/9  "GIState"
  Gateway_States/10 -> Bus Creator/11  "GatewayClearanceAI"
  Gateway_States/12 -> Bus Creator/12  "GatewayClearanceEBI"
  Gateway_States/11 -> Bus Creator/13  "GatewayClearanceSI"
  Gateway_States/9 -> Bus Creator/17  "PDIState"
  Gateway_States/5 -> Bus Creator/8  "EBIState"
  Gateway_States/1 -> Bus Creator/6  "CRC"
  Gateway_States/15 -> Bus Creator/3  "AngleGradientLimitationSI"
  Gateway_States/7 -> Bus Creator/18  "SIState"
  Gateway_States/13 -> Bus Creator/14  "LimitationsReceivedSI"
  Gateway_States/17 -> Bus Creator/19  "THIState"
  Gateway_States/19 -> Bus Creator/15  "MsgTimeoutDisplay"
  Gateway_States/8 -> Bus Creator/20  "VIState"

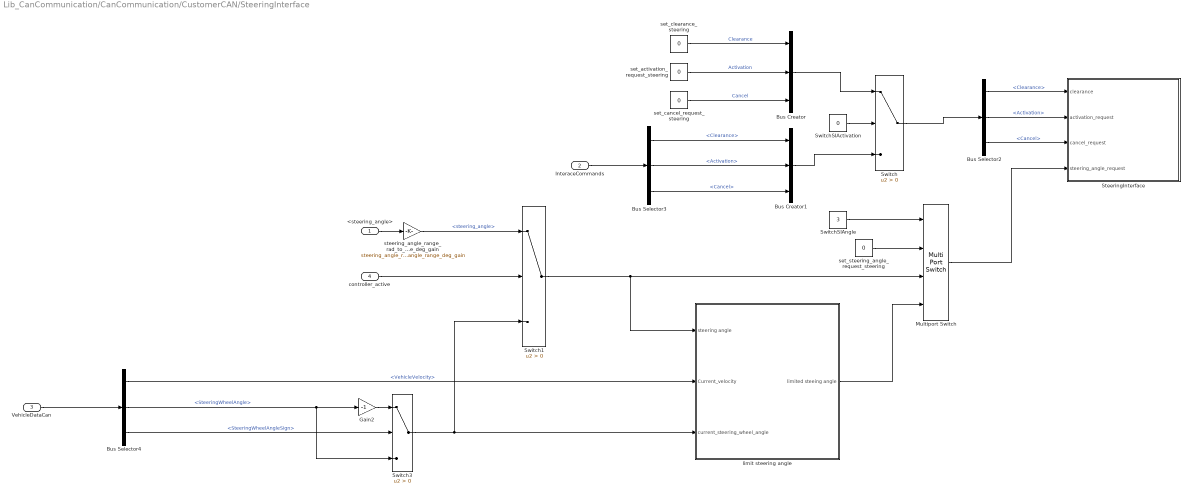
== system Lib_CanCommunication/CanCommunication/CustomerCAN/SteeringInterface ==
  <steering_angle> : Inport
  InteraceCommands : Inport  Port=2
  VehicleDataCan : Inport  Port=3
  controller_active : Inport  Port=4
  Bus Creator : BusCreator  Inputs=3
  Bus Creator1 : BusCreator  Inputs=3
  Bus Selector2 : BusSelector  OutputSignals=Clearance,Activation,Cancel
  Bus Selector3 : BusSelector  OutputSignals=SteeringInterfaceCommands.Clearance,SteeringInterfaceCommands.Activation,SteeringInterfaceCommands.Cancel
  Bus Selector4 : BusSelector  OutputSignals=Motion.VehicleVelocity,Steering.SteeringWheelAngle,Steering.SteeringWheelAngleSign
  Gain2 : Gain  Gain=-1
  Multiport Switch : MultiPortSwitch
  SteeringInterface : Subsystem
  Switch : Switch  Criteria=u2 > Threshold
  Switch1 : Switch  Criteria=u2 > Threshold
  Switch3 : Switch  Criteria=u2 > Threshold
  SwitchSIActivation : Constant  Value=0
  SwitchSIAngle : Constant  Value=3
  limit steering angle : Subsystem
  set_activation_request_steering : Constant  Value=0  OutDataTypeStr=boolean
  set_cancel_request_steering : Constant  Value=0  OutDataTypeStr=boolean
  set_clearance_steering : Constant  Value=0  OutDataTypeStr=uint8
  set_steering_angle_request_steering : Constant  Value=0
  steering_angle_range_rad_to_steering_wheel_angle_range_deg_gain : Gain  Gain=steering_angle_range_rad_to_steering_wheel_angle_range_deg_gain
  wires:
  VehicleDataCan/1 -> Bus Selector4/1
  Switch3/1 -> limit steering angle/3(current_steering_wheel_angle), Switch1/3
  Bus Selector4/1 -> limit steering angle/2(Current_velocity)  "<VehicleVelocity>"
  Bus Selector4/3 -> Switch3/2  "<SteeringWheelAngleSign>"
  Bus Selector4/2 -> Gain2/1, Switch3/3  "<SteeringWheelAngle>"
  Gain2/1 -> Switch3/1
  controller_active/1 -> Switch1/2
  steering_angle_range_rad_to_steering_wheel_angle_range_deg_gain/1 -> Switch1/1  "<steering_angle>"
  Switch1/1 -> Multiport Switch/3, limit steering angle/1(steering angle)
  InteraceCommands/1 -> Bus Selector3/1
  SwitchSIActivation/1 -> Switch/2
  Bus Creator/1 -> Switch/1
  SwitchSIAngle/1 -> Multiport Switch/1
  Multiport Switch/1 -> SteeringInterface/4(steering_angle_request)
  Bus Selector3/1 -> Bus Creator1/1  "<Clearance>"
  set_clearance_steering/1 -> Bus Creator/1  "Clearance"
  set_cancel_request_steering/1 -> Bus Creator/3  "Cancel"
  set_activation_request_steering/1 -> Bus Creator/2  "Activation"
  Bus Selector3/3 -> Bus Creator1/3  "<Cancel>"
  Bus Selector3/2 -> Bus Creator1/2  "<Activation>"
  limit steering angle/1(limited steeing angle) -> Multiport Switch/4
  Bus Creator1/1 -> Switch/3
  Bus Selector2/1 -> SteeringInterface/1(clearance)  "<Clearance>"
  Bus Selector2/3 -> SteeringInterface/3(cancel_request)  "<Cancel>"
  Bus Selector2/2 -> SteeringInterface/2(activation_request)  "<Activation>"
  Switch/1 -> Bus Selector2/1
  <steering_angle>/1 -> steering_angle_range_rad_to_steering_wheel_angle_range_deg_gain/1
  set_steering_angle_request_steering/1 -> Multiport Switch/2

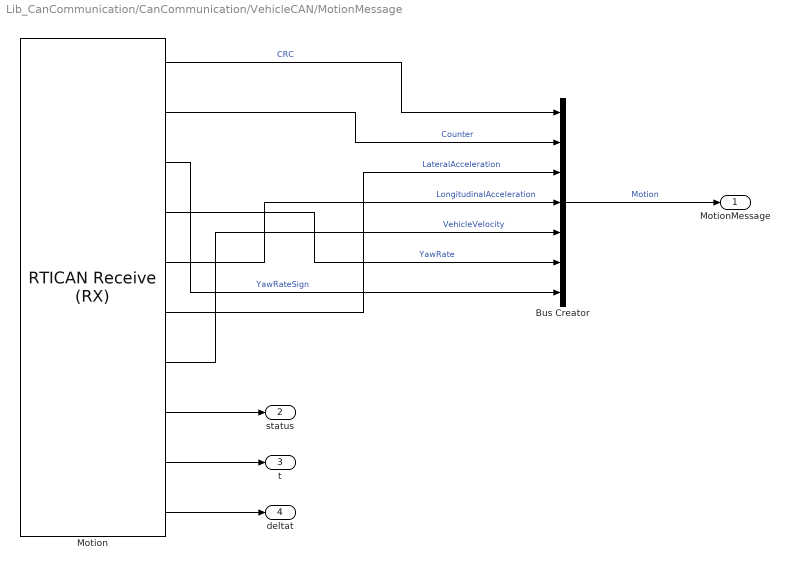
== system Lib_CanCommunication/CanCommunication/VehicleCAN/MotionMessage ==
  Bus Creator : BusCreator  Inputs=CRC,Counter,LateralAcceleration,LongitudinalAcceleration,VehicleVelocity,YawRate,YawRateSign  OutDataTypeStr=Bus: Motion  NonVirtualBus=on
  Motion : rtican/RTICAN Receive (RX)   Reserved1=[]  Reserved2=[]  Reserved3=[]  Reserved4=[]  SfcnMessage=[]  Msg_Struct=[]  BoardTypeNo=[]  BoardNo=[]  ChannelNo=[]  Parameters=[]  DialogFcn=[]  UnitName=[]  Revision=[]  UnitValues=[]  DSProperties=struct('RTI',struct('Version',uint32(5),'BlockType',struct('isSLSource',uint8(1),'isSLSink',uint8(1),'isHWSource',uint8(0),'isHWSink',uint8(0),'isSetup',uint8(0),'isInline',uint8(1),'isNonInline',uint8(0),'isInterrupt',uint8(0),'isChannelwise',uint8(0)),'IOBoardType','RTICAN','UnitType','MESSAGE','Identifier','RX','DialogType','MSVC','BlockSet','RTICAN','SlaveProcessor','CAN'))  RTIBlockInterface=struct('OutputPortsWidth',int32([1 1 1 1 1 1 1 1 1 1]),'OutputPortsActive',[1 1 1 1 1 1 1 1 1 1],'OutputPortsName',{{'CRC','Counter','YawRateSign','YawRate','LongitudinalAcceleration','LateralAcceleration','VehicleVelocity',['RX status'],['RX time'],['RX delta time']}},'OutputPortsDataType',{{'SS_UINT8','SS_UINT8','SS_BOOLEAN','SS_DOUBLE','SS_DOUBLE','SS_DOUBLE','SS_DOUBLE','SS_DOUBLE','SS_DOUBLE','SS_DOUBLE'}},'OutputPortsLabel',{{'CRC','Counter','YawRateSign','YawRate','LongitudinalAcceleration','LateralAcceleration','VehicleVelocity','','',''}},'OutputPortsLabelMode','ON','InputPortsWidth',int32(0),'InputPortsActive',0,'DialogFcn','rtican_message_interface_gui','BlockDisplay',{{'','center'}},'IconTransparency','on','ParameterTunableNames',{{}},'InitLevel',3,'BlockName',struct('Token',{{'Motion'}}),'SampleTime',{{-1}},'TriggerPort',{{'none'}},'EnablePort',{{'none'}})  RTIBlockParameters="struct('BoardTypeNo',{{1,'OFF',[]}},'BoardNo',{{1,'ON',[1 16]}},'ChannelNo',{{2,'ON',[1 2]}},'Parameters',{{struct('DataFileSupport',struct('DataFileSelectedMaster',1,'DataFileSelectedLocal',0,'DataFileName','c:\\users\\esterle\\documents\\repositories\\stack\\src\\autobox\\simulink\\dbc\\vehicledata_can_tfd7-17008-03_fortiss_gte.dbc|','DataFileDate',{{{['06-Jul-2018 10:05:43']},{['06-Jul-2018 10:06:03']}}},'SelectedFile',['<no file selected>']),'Options',struct('StatusSelected',1,'TimeSelected',1,'DeltaTimeSelected',1,'BytePortSelected',0,'MessageLengthSelected',0,'TriggerPort',struct('Selected',0,'TriggerType',0),'UserCoding',struct('Selected',0,'InterfaceFile','UserDecodingFile','FcnName','UserDecodeFcn','InportSelected',0,'InportWidth',1,'OutportSelected',0,'OutportWidth',1),'EnablePortSelected',0,'SignalOnPortnameSelected',1,'UseRXService',0),'Message',struct('MsgOnBlocknameSelected',1,'MsgName','Motion','MsgIdFormat',0,'MsgId',1,'MsgLength',8,'NumSignals',7,'SampleTime',-1,'Signal',struct('SgnName',{'CRC','Counter','YawRateSign','YawRate','LongitudinalAcceleration','LateralAcceleration','VehicleVelocity'},'SgnStartBit',{0,8,12,16,30,40,48},'SgnLength',{8,4,1,14,10,8,16},'SgnType',{0,0,0,0,0,0,0},'ModeValue',{-1,-1,-1,-1,-1,-1,-1},'DataType',{0,0,0,0,0,0,0},'ByteLayout',{0,0,0,0,0,0,0},'Factor',{1,1,1,0.01,2^-5,0.01,0.01},'Offset',{0,0,0,0,-16,-1.27,0},'SgnComment',{{['Checksum for Motion message:  CRC = Byte1 XOR Byte2 XOR Byte3 XOR Byte4 XOR Byte5 XOR Byte6 XOR Byte7. ']},{['Counter for Motion message, incremented with every transmittal and periodically running from 0 to 15.']},{['Sign of the yaw rate of the ego vehicle. ']},{['Yaw rate of the ego vehicle.']},{['Longitudinal acceleration of the ego vehicle.']},{['Lateral acceleration of ego vehicle. A negative sign indicates accelerations to the right. ']},{['Velocity of the ego vehicle. ']}},'SgnUnit',{'-','-','-','deg/s','m/s²','g','km/h'},'Min',{0,0,0,0,-16,-1.27,0},'Max',{255,15,1,163.82,15.90625,1.27,655.32},'SLDataType',{'SS_UINT8','SS_UINT8','SS_BOOLEAN','SS_DOUBLE','SS_DOUBLE','SS_DOUBLE','SS_DOUBLE'}),'MsgIdNumFormat',0,'MsgComment',{{['Dynamic vehicle data. ']}}),'Version',1.2,'general',struct('isFromLib',0)),'OFF',[]}},'GroupId',{{struct('Group',{{'RTICAN'}},'No',1,'Behavior',{{'NAMECHANGE'}},'BlockType',{{'SINK'}},'NameChangeFlag',0),'OFF',[]}},'SFcnRTICANMessage',{{struct('MsgType','RX','SFcnPortType','Scalar','MsgName','Motion','MsgIdFormat','STD','MsgId',1,'MsgLength',8,'NumSignals',7,'SampleTime',-1,'Signal',struct('SgnName',{'CRC','Counter','YawRateSign','YawRate','LongitudinalAcceleration','LateralAcceleration','VehicleVelocity'},'SgnStartBit',{0,8,12,16,30,40,48},'SgnLength',{8,4,1,14,10,8,16},'SgnType',{'standard','standard','standard','standard','standard','standard','standard'},'ModeValue',{-1,-1,-1,-1,-1,-1,-1},'DataType',{['unsigned int'],['unsigned int'],['unsigned int'],['unsigned int'],['unsigned int'],['unsigned int'],['unsigned int']},'ByteLayout',{['little endian'],['little endian'],['little endian'],['little endian'],['little endian'],['little endian'],['little endian']},'Factor',{1,1,1,0.01,2^-5,0.01,0.01},'Offset',{0,0,0,0,-16,-1.27,0},'SLDataType',{'SS_UINT8','SS_UINT8','SS_BOOLEAN','SS_DOUBLE','SS_DOUBLE','SS_DOUBLE','SS_DOUBLE'}),'StatusSelected','yes','TimeSelected','yes','DeltaTimeSelected','yes','BytePortSelected','no','MessageLengthSelected','no','TriggerPort',struct('Selected','no','TriggerType',0),'UserCoding',struct('Selected','no','InterfaceFile','UserDecodingFile','FcnName','UserDecodeFcn','InportSelected','no','InportWidth',1,'OutportSelected','no','OutportWidth',1),'EnablePortSelected','no','UseRXService','no','BoardType','DS1','BoardNo',1,'ControllerNo',1),'OFF',[]}},'TLCFileName',{{'rtican_rx_message','OFF',[]}})"  RTISFcnParameters=struct('SFcnRTICANMessage','struct','TLCFileName','char')  RTIBlockParaDefault=struct('BoardTypeNo',4302,'BoardNo',1,'ChannelNo',1,'Parameters',struct('DataFileSupport',struct('DataFileSelectedMaster',0,'DataFileSelectedLocal',0,'DataFileName','','DataFileDate','','SelectedFile',['<no file selected>']),'Options',struct('StatusSelected',1,'TimeSelected',1,'DeltaTimeSelected',1,'BytePortSelected',0,'MessageLengthSelected',0,'TriggerPort',struct('Selected',0,'TriggerType','rising'),'UserCoding',struct('Selected',0,'InterfaceFile','UserDecodingFile','FcnName','UserDecodeFcn','InportSelected',0,'InportWidth',1,'OutportSelected',0,'OutportWidth',1),'EnablePortSelected',0,'SignalOnPortnameSelected',1,'UseRXService',0),'Message',struct('MsgOnBlocknameSelected',0,'MsgName',['RX Message'],'MsgIdFormat',0,'MsgId',100,'MsgLength',8,'NumSignals',1,'SampleTime',-1,'Signal',struct('SgnName',['RX signal'],'SgnStartBit',0,'SgnLength',8,'SgnType',0,'ModeValue',-1,'DataType',0,'SLDataType','SS_DOUBLE','ByteLayout',0,'Factor',1,'Offset',0,'Min',0,'Max',255,'SgnComment',{{}},'SgnUnit',''),'MsgIdNumFormat',0,'MsgComment',{{''}}),'Version',1.2,'general',struct('isFromLib',1)),'GroupId',struct('Group',{{'RTICAN'}},'No',1,'Behavior',{{'NAMECHANGE'}},'BlockType',{{'SINK'}},'NameChangeFlag',0),'SFcnRTICANMessage',struct('MsgType','RX','MsgName',['RX Message'],'MsgIdFormat','STD','MsgId',100,'MsgLength',8,'NumSignals',1,'SampleTime',-1,'Signal',struct('SgnName',['RX signal'],'SgnStartBit',0,'SgnLength',8,'SgnType','standard','ModeValue',-1,'DataType',['unsigned int'],'ByteLayout',['little endian'],'SLDataType','SS_DOUBLE','Factor',1,'Offset',0),'StatusSelected','yes','TimeSelected','yes','DeltaTimeSelected','yes','BytePortSelected','no','MessageLengthSelected','no','EnablePortSelected','no','UserCoding',struct('Selected','no','InterfaceFile','UserDecodingFile','FcnName','UserDecodeFcn','InportSelected','no','InportWidth',1,'OutportSelected','no','OutportWidth',1),'TriggerPort',struct('Selected','no','TriggerType','rising'),'UseRXService','no','BoardType','DS4302','BoardNo',1,'ControllerNo',1,'SFcnPortType','Scalar'),'TLCFileName','rtican_rx_message')
      settings: AttributesFormatString=Group Id: RTICAN1\n  SourceProductName=dSPACE RTI CAN Blockset
  MotionMessage : Outport  VectorParamsAs1DForOutWhenUnconnected=off
  status : Outport  Port=2  VectorParamsAs1DForOutWhenUnconnected=off
  t : Outport  Port=3  VectorParamsAs1DForOutWhenUnconnected=off
  deltat : Outport  Port=4  VectorParamsAs1DForOutWhenUnconnected=off
  wires:
  Motion/10 -> deltat/1
  Motion/8 -> status/1
  Motion/9 -> t/1
  Bus Creator/1 -> MotionMessage/1  "Motion"
  Motion/2 -> Bus Creator/2  "Counter"
  Motion/1 -> Bus Creator/1  "CRC"
  Motion/6 -> Bus Creator/3  "LateralAcceleration"
  Motion/5 -> Bus Creator/4  "LongitudinalAcceleration"
  Motion/7 -> Bus Creator/5  "VehicleVelocity"
  Motion/4 -> Bus Creator/6  "YawRate"
  Motion/3 -> Bus Creator/7  "YawRateSign"
